simulink model "robusni_lin_regulacija_nelin_sim"  (R2020a)
settings: Solver=ode5  StartTime=0.0  StopTime=tfin  FixedStep=1e-4  RelTol=1e-3
values from neighbouring files (symbols this model uses):
  disturb_X = 0.2*Xe    (= 0.978133730754)    [sum_lin_regulacija_nelin_sim_matlab.m]
  F_lower_limit = 0    [sum_lin_regulacija_nelin_sim_matlab.m]
  F_upper_limit = 1e-3*Fe    (= 0.00320891060125)    [sum_lin_regulacija_nelin_sim_matlab.m]
  Fe = 3.20891060125344    (= 3.20891060125)    [sum_lin_regulacija_nelin_sim_matlab.m]
  K1 = 0.03    [sum_lin_regulacija_nelin_sim_matlab.m]
  K2 = 0.5    [sum_lin_regulacija_nelin_sim_matlab.m]
  Kc1 = 1/abs(freqresp((1+1/Ti1/s)*G_design,w1_design))    [sum_lin_regulacija_nelin_sim_matlab.m]
  mi_max = 1    [sum_lin_regulacija_nelin_sim_matlab.m]
  S_step1 = delta    (= 0)    [sum_lin_regulacija_nelin_sim_matlab.m]
  S_step2 = delta    (= 0)    [sum_lin_regulacija_nelin_sim_matlab.m]
  S_time_step1 = 5    [sum_lin_regulacija_nelin_sim_matlab.m]
  S_time_step2 = 40    [sum_lin_regulacija_nelin_sim_matlab.m]
  Se = 0.218662692463450    (= 0.218662692463)    [sum_lin_regulacija_nelin_sim_matlab.m]
  SF = 10    [sum_lin_regulacija_nelin_sim_matlab.m]
  std_noise = 1e-5*Se    (= 2.18662692463e-06)    [sum_lin_regulacija_nelin_sim_matlab.m]
  V = 4    [sum_lin_regulacija_nelin_sim_matlab.m]
  x10 = X_initial    (= 4.88375)    [sum_lin_regulacija_nelin_sim_matlab.m]
  x20 = S_initial    (= 0.2325)    [sum_lin_regulacija_nelin_sim_matlab.m]
  Y = Ynom    (= 0.5)    [sum_lin_regulacija_nelin_sim_matlab.m]
undefined symbols (not defined in the file or in its folder): magnitude
libraries: cstblocks x2
settings Model: Creator=anaMceranic  LastModifiedBy=anaMceranic
settings DataIOCC: ReturnWorkspaceOutputs=off

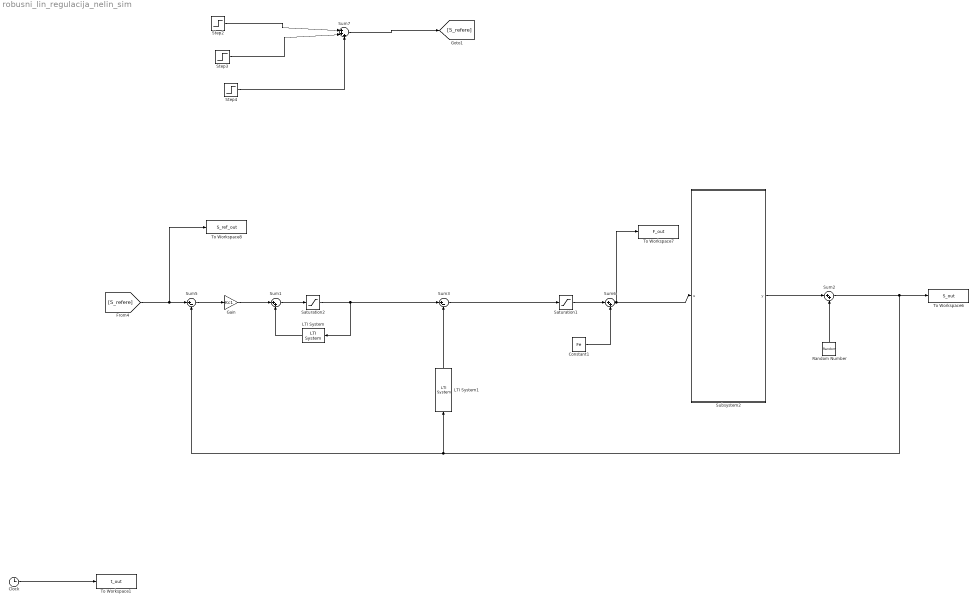
== system robusni_lin_regulacija_nelin_sim ==
  Clock : Clock
  Constant1 : Constant  Value=Fe
  Gain : Gain  Gain=Kc1
  LTI System : cstblocks/LTI System  sys=KPI_aw  IC=[]
  LTI System1 : cstblocks/LTI System  sys=Kfb  IC=[]
  Random Number : RandomNumber  Variance=std_noise  SampleTime=0.1
  Saturation1 : Saturate  UpperLimit=F_upper_limit  LowerLimit=F_lower_limit
  Saturation2 : Saturate  UpperLimit=F_upper_limit  LowerLimit=F_lower_limit
  Step2 : Step  Time=0  Before=Se  After=Se  SampleTime=0
  Step3 : Step  Time=S_time_step1  After=S_step1  SampleTime=0
  Step4 : Step  Time=S_time_step2  After=-S_step2  SampleTime=0
  Subsystem2 : Subsystem
  Sum1 : Sum  Inputs=|++
  Sum2 : Sum  Inputs=|++
  Sum3 : Sum  Inputs=|+-
  Sum5 : Sum  Inputs=|+-
  Sum6 : Sum  Inputs=|++
  Sum7 : Sum  Inputs=|+++
  To Workspace1 : ToWorkspace  VariableName=t_out  SampleTime=-1
  To Workspace6 : ToWorkspace  VariableName=S_out  SampleTime=-1
  To Workspace7 : ToWorkspace  VariableName=F_out  SampleTime=-1
  To Workspace8 : ToWorkspace  VariableName=S_ref_out  SampleTime=-1
  wires:
  Clock/1 -> To Workspace1/1
  Sum6/1 -> To Workspace7/1, Subsystem2/1(u)
  Saturation1/1 -> Sum6/1
  Constant1/1 -> Sum6/2
  Sum5/1 -> Gain/1
  Sum7/1 -> [S_refere]
  Step2/1 -> Sum7/1
  [S_refere] -> To Workspace8/1, Sum5/1
  Gain/1 -> Sum1/1
  Sum1/1 -> Saturation2/1
  LTI System/1 -> Sum1/2
  Step3/1 -> Sum7/2
  Step4/1 -> Sum7/3
  Subsystem2/1(y) -> Sum2/1
  Sum2/1 -> Sum5/2, LTI System1/1, To Workspace6/1
  Random Number/1 -> Sum2/2
  Saturation2/1 -> Sum3/1, LTI System/1
  Sum3/1 -> Saturation1/1
  LTI System1/1 -> Sum3/2

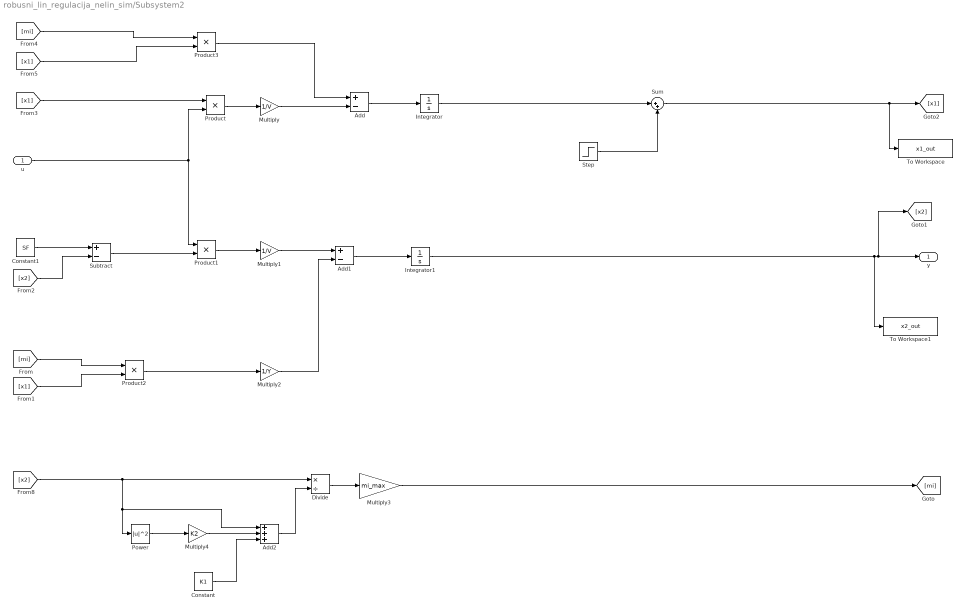
== system robusni_lin_regulacija_nelin_sim/Subsystem2 ==
  u : Inport
  Add : Sum  Inputs=+-
  Add1 : Sum  Inputs=+-
  Add2 : Sum  Inputs=+++
  Constant : Constant  Value=K1
  Constant1 : Constant  Value=SF
  Divide : Product  Inputs=*/
  Integrator : Integrator  InitialCondition=x10
  Integrator1 : Integrator  InitialCondition=x20
  Multiply : Gain  Gain=1/V
  Multiply1 : Gain  Gain=1/V
  Multiply2 : Gain  Gain=1/Y
  Multiply3 : Gain  Gain=mi_max
  Multiply4 : Gain  Gain=K2
  Power : Math  Operator=magnitude^2  SaturateOnIntegerOverflow=on
  Product{,1..3} (4 alike) : Product
  Step : Step  Time=2  After=disturb_X  SampleTime=0
  Subtract : Sum  Inputs=+-
  Sum : Sum  Inputs=|++
  To Workspace : ToWorkspace  VariableName=x1_out  SampleTime=-1
  To Workspace1 : ToWorkspace  VariableName=x2_out  SampleTime=-1
  y : Outport
  wires:
  [x1] -> Product2/2
  Product2/1 -> Multiply2/1
  Multiply/1 -> Add/2
  Add2/1 -> Divide/2
  Constant/1 -> Add2/3
  [x1] -> Product3/2
  Multiply4/1 -> Add2/2
  [mi] -> Product2/1
  Multiply3/1 -> [mi]
  Power/1 -> Multiply4/1
  Constant1/1 -> Subtract/1
  [x2] -> Subtract/2
  Add1/1 -> Integrator1/1
  Multiply2/1 -> Add1/2
  Integrator1/1 -> [x2], y/1, To Workspace1/1
  Divide/1 -> Multiply3/1
  Product3/1 -> Add/1
  u/1 -> Product1/1, Product/2
  [x1] -> Product/1
  Multiply1/1 -> Add1/1
  Product1/1 -> Multiply1/1
  Subtract/1 -> Product1/2
  [x2] -> Divide/1, Add2/1, Power/1
  Add/1 -> Integrator/1
  Product/1 -> Multiply/1
  [mi] -> Product3/1
  Integrator/1 -> Sum/1
  Sum/1 -> To Workspace/1, [x1]
  Step/1 -> Sum/2
